simulink model "ovap_sim"  (R2025a)
settings: Solver=FixedStepAuto  StartTime=0.0  StopTime=100  FixedStep=0.002  RelTol=1e-3
undefined symbols (not defined in the file): X, Y, Z
libraries: sm_lib x88, nesl_utility x45, simulink_extras x31, slpidlib x8
(part 4 of 5)

== matlab function ovap_sim/3_Actuator_Dynamics/MATLAB Function ==
  settings: updateMethod=DISCRETE  sampleTime=0.002
  data: cmd_thrust input; phys_thrust output; cmd_alpha input; cmd_beta input; dt input; tau_motor input; tau_servo input; rate_lim input; lim_tilt input; phys_alpha output; phys_beta output
function [phys_thrust, phys_alpha, phys_beta] = Actuator_Dynamics(cmd_thrust, cmd_alpha, cmd_beta, ...
    dt, tau_motor, tau_servo, rate_lim, lim_tilt)
% =========================================================================
% Tên hàm: Actuator_Dynamics (Động lực học Cơ cấu chấp hành)
% Chức năng: Đóng vai trò làm "Bộ lọc Hiện thực". Biến các mệnh lệnh toán học
%            tức thời (cmd_) thành phản ứng vật lý thực tế có độ trễ (phys_).
% Nguyên lý: Mô phỏng Quán tính Rotor (First-Order Lag) và Giới hạn bánh răng
%            Servo (Rate Limit & Saturation).
% =========================================================================

    % ---------------------------------------------------------------------
    % 1. BỘ NHỚ VẬT LÝ (PERSISTENT STATE)
    % Ý nghĩa: Trong thế giới thực, một vật thể không thể dịch chuyển tức thời
    % từ trạng thái A sang B. Trạng thái tiếp theo luôn phụ thuộc vào trạng
    % thái hiện tại. Biến persistent đóng vai trò là "quán tính" của hệ thống.
    % ---------------------------------------------------------------------
    persistent prev_thrust prev_alpha prev_beta
    
    % Khởi tạo trạng thái đứng im khi bắt đầu bật điện (t = 0)
    if isempty(prev_thrust)
        prev_thrust = zeros(8,1); % Lực đẩy 8 motor = 0 N
        prev_alpha  = zeros(4,1); % Góc gật 4 ngàm = 0 rad
        prev_beta   = zeros(4,1); % Góc lật 4 ngàm = 0 rad
    end

    % ---------------------------------------------------------------------
    % 2. ĐỘNG LỰC HỌC ĐỘNG CƠ (MOTOR DYNAMICS - THUẬT TOÁN PT1)
    % Bản chất: Lõi chuông motor và cánh quạt 7-inch có khối lượng (Inertia).
    % Khi ESC bơm dòng điện, từ trường sinh ra momen xoắn để thắng sức ỳ này.
    % Thời gian để đạt được lực đẩy yêu cầu được đặc trưng bởi tau_motor (Ví dụ: 0.03s).
    % ---------------------------------------------------------------------
    % Tính hệ số lọc (Alpha) của bộ lọc thông thấp bậc 1 (First-Order Low-pass)
    % Hệ số này quyết định motor "bám theo" lệnh nhanh hay chậm dựa trên bước nhảy dt.
    alpha_m = dt / (tau_motor + dt);
    
    % Lực đẩy thực tế sẽ bám đuổi (chasing) lệnh yêu cầu.
    % Nếu lệch càng nhiều (cmd - prev lớn), motor tăng tốc càng mạnh.
    thrust_next = prev_thrust + alpha_m * (cmd_thrust - prev_thrust);
    
    % Giới hạn vật lý: Động cơ BLDC gắn cánh quạt tĩnh không thể tạo lực đẩy âm
    % (Trừ khi ESC dùng chế độ 3D đảo chiều quay, nhưng OVAP-X1 không dùng).
    phys_thrust = max(0, thrust_next); 

    % ---------------------------------------------------------------------
    % 3. ĐỘNG LỰC HỌC SERVO (SERVO DYNAMICS - LAG & RATE LIMIT)
    % Bản chất: Servo xịn như KST có mạch điều khiển bên trong (gây trễ tau_servo),
    % và hộp số bánh răng kim loại có tốc độ quay tối đa (rate_lim, ví dụ: 300 deg/s).
    % ---------------------------------------------------------------------
    % Hệ số độ trễ của mạch điện điều khiển Servo
    alpha_s = dt / (tau_servo + dt);
    
    % GIỚI HẠN TỐC ĐỘ (Rate Limit): Quãng đường góc lớn nhất (rad) mà bánh răng 
    % cơ khí có thể quét được trong khoảng thời gian siêu ngắn dt (0.002s).
    max_step = rate_lim * dt; 
    
    % ================= KÊNH ALPHA (NGÀM GẬP PITCH) =================
    % 3.1. Tính vị trí lý tưởng mà Servo "muốn" đạt tới (chỉ xét độ trễ mạch điện)
    ideal_alpha = prev_alpha + alpha_s * (cmd_alpha - prev_alpha); 
    
    % 3.2. Tính quãng đường góc cần di chuyển trong bước này
    delta_alpha = ideal_alpha - prev_alpha;
    
    % 3.3. ÁP DỤNG NÚT THẮT CỔ CHAI CƠ KHÍ (Rate Clamping)
    % Nếu lệnh bắt Servo quay nhanh hơn khả năng của motor bên trong, 
    % nó sẽ bị "nghẽn" lại và chỉ xoay được đúng bằng max_step.
    delta_alpha = max(min(delta_alpha, max_step), -max_step);      
    
    % 3.4. Vị trí thực tế Servo đạt được sau 1 bước dt
    phys_alpha = prev_alpha + delta_alpha;
    
    % 3.5. VA CHẠM CƠ KHÍ (Hard Stop / Saturation)
    phys_alpha = max(min(phys_alpha, lim_tilt), -lim_tilt);        
    
    % ================= KÊNH BETA (NGÀM LẬT ROLL) =================
    % (Áp dụng chính xác các quy luật vật lý tương tự như Kênh Alpha)
    ideal_beta = prev_beta + alpha_s * (cmd_beta - prev_beta);     
    delta_beta = ideal_beta - prev_beta;
    delta_beta = max(min(delta_beta, max_step), -max_step);        
    
    phys_beta = prev_beta + delta_beta;
    phys_beta = max(min(phys_beta, lim_tilt), -lim_tilt);          

    % ---------------------------------------------------------------------
    % 4. CẬP NHẬT TRẠNG THÁI (TIME MARCHING)
    % Ý nghĩa: Dòng thời gian trôi đi. Hiện tại của vòng lặp này sẽ trở thành 
    % quá khứ (prev_) cho vòng lặp tích phân tiếp theo.
    % ---------------------------------------------------------------------
    prev_thrust = phys_thrust;
    prev_alpha  = phys_alpha;
    prev_beta   = phys_beta;
end

== matlab function ovap_sim/2_Flight_Control_System/PID - 1/MATLAB Function1 ==
  data: ax_world input; cmd_hw_alpha output; ay_world input; cmd_thrust_z input; cmd_effort_roll input; cmd_effort_pitch input; cmd_effort_yaw input; yaw input; pitch input; roll input; phys_alpha_hw input; phys_beta_hw input; m input; g input; dir_alpha input; dir_beta input; lim_alpha input; lim_beta input; cmd_hw_beta output; cmd_thrust output; R_mat input; eta_c input; lam_c input; c_q input; dir_top input; max_thrust input
function [cmd_hw_alpha, cmd_hw_beta, cmd_thrust] = OVAP_Unified_Mixer(...
    ax_world, ay_world, ...                             
    cmd_thrust_z, cmd_effort_roll, cmd_effort_pitch, cmd_effort_yaw, ... 
    yaw, pitch, roll, ...                               
    phys_alpha_hw, phys_beta_hw, ...                    
    m, g, ...                                           
    dir_alpha, dir_beta, lim_alpha, lim_beta, ...
    R_mat, eta_c, lam_c, c_q, dir_top, max_thrust)            
% =========================================================================
% BỘ ĐIỀU KHIỂN CHẤP HÀNH TỔNG HỢP OVAP (UNIFIED ACTUATION MIXER) V7.5
% Kiến trúc: SYNCHRONOUS VECTORING + FEEDFORWARD ATTITUDE ASSIST
% [CẬP NHẬT MỚI]: Auto-Routing dựa trên Tọa độ Ma trận Hình học (R_mat).
% =========================================================================
    
    phys_alpha_hw = phys_alpha_hw(:); 
    phys_beta_hw  = phys_beta_hw(:);
    dir_alpha     = dir_alpha(:);
    dir_beta      = dir_beta(:);
    dir_top       = dir_top(:); 
    
    % =====================================================================
    % [HỆ SỐ HỖ TRỢ TƯ THẾ (FEEDFORWARD GAINS)]
    % =====================================================================
    K_assist_pitch = 0; 
    K_assist_roll  = 0; 
    lim_assist     = 0.17; 
    
    % =====================================================================
    % [TRIGGER BÁN CẦU] - NHẬN DIỆN MÁY BAY LẬT ÚP
    % =====================================================================
    inv_x = sign(cos(pitch) + eps);  
    inv_y = sign(cos(roll)  + eps);
    
    % =====================================================================
    % PHÂN VÙNG 1: ĐỒNG BỘ PHẢN HỒI (HARDWARE TO MATH)
    % =====================================================================
    math_alpha_fb = phys_alpha_hw ./ dir_alpha;  
    math_beta_fb  = phys_beta_hw  ./ dir_beta;  
    
    % =====================================================================
    % PHÂN VÙNG 2: BỘ TÍNH TOÁN VỊ TRÍ & TÍCH HỢP HỖ TRỢ TƯ THẾ
    % =====================================================================
    ax_heading = ax_world * cos(yaw) + ay_world * sin(yaw);   
    ay_heading = -ax_world * sin(yaw) + ay_world * cos(yaw); 
    
    ax_body_sync = ax_heading; 
    ay_body_sync = ay_heading; 
    
    ratio_x = max(min(ax_body_sync / g, 0.99), -0.99); 
    ratio_y = max(min(ay_body_sync / g, 0.99), -0.99); 
    
    alpha_base_array = zeros(4,1) + asin(ratio_x);
    beta_base_array  = zeros(4,1) + asin(ratio_y);  
    
    assist_pitch = max(min(cmd_effort_pitch * K_assist_pitch, lim_assist), -lim_assist);
    assist_roll  = max(min(cmd_effort_roll  * K_assist_roll,  lim_assist), -lim_assist);
    
    cmd_math_alpha = alpha_base_array + pitch + assist_pitch; 
    cmd_math_beta  = beta_base_array  - roll  + assist_roll;  
    
    cmd_math_alpha = atan2(sin(cmd_math_alpha), cos(cmd_math_alpha));
    cmd_math_beta  = atan2(sin(cmd_math_beta),  cos(cmd_math_beta));
    
    % =====================================================================
    % PHÂN VÙNG 3: BỘ PHÂN BỔ NGÀM VẬT LÝ (HARDWARE SERVO MAPPER)
    % =====================================================================
    cmd_hw_alpha = cmd_math_alpha .* dir_alpha; 
    cmd_hw_beta  = cmd_math_beta  .* dir_beta;  
    
    cmd_hw_alpha = max(min(cmd_hw_alpha, lim_alpha), -lim_alpha); 
    cmd_hw_beta  = max(min(cmd_hw_beta,  lim_beta),  -lim_beta);  
    
    % =====================================================================
    % PHÂN VÙNG 4: BỘ TRỘN ĐỘNG CƠ (R-CRM MOTOR MIXER TƯỜNG MINH)
    % =====================================================================
    global_alpha = math_alpha_fb - pitch;  
    global_beta  = math_beta_fb  + roll;
    
    mean_global_alpha = mean(abs(global_alpha)); 
    mean_global_beta  = mean(abs(global_beta));  
    
    total_z_req = cmd_thrust_z + m * g;
    T_base = (total_z_req / (cos(mean_global_alpha) * cos(mean_global_beta))) / 4;
    
    K_cross_pitch = 0.0; 
    K_cross_roll = 0.0; 
    pitch_parasitic = K_cross_pitch * sin(mean(math_alpha_fb)); 
    roll_parasitic  = K_cross_roll  * sin(mean(math_beta_fb));  
    
    real_cmd_pitch = (cmd_effort_pitch - pitch_parasitic) * inv_x;
    real_cmd_roll  = (cmd_effort_roll  - roll_parasitic)  * inv_y;
    
    % [CẬP NHẬT]: Trích xuất dist_x, dist_y (Vẫn lấy từ R_mat để dễ chỉnh kích thước)
    dist_x = abs(R_mat(1, 1));
    dist_y = abs(R_mat(1, 2));
    
    d_pitch = real_cmd_pitch / (4 * dist_x);
    d_roll  = real_cmd_roll  / (4 * dist_y);
    d_yaw   = cmd_effort_yaw / 4; 
    
    cmd_thrust = zeros(8,1); 
    limit_thrust = max_thrust(end);

    % -------------------------------------------------------------------------
    % ARM 1: FRONT-RIGHT (FR) 
    % Gốc: math_thrust(1) = base + pitch - roll + yaw (Top)
    %      math_thrust(6) = base + pitch - roll - yaw (Bot)
    % -------------------------------------------------------------------------
    T_arm1  = T_base + d_pitch - d_roll;
    dT_1    = d_yaw / c_q; % Dấu dương để T_top tăng (+yaw), T_bot giảm (-yaw)
    
    T_bot_6 = (T_arm1 - dT_1) / (eta_c + lam_c);
    T_top_1 = T_arm1 - eta_c * T_bot_6;
    
    if T_bot_6 < 0, T_bot_6 = 0; T_top_1 = T_arm1; end
    if T_top_1 < 0, T_top_1 = 0; T_bot_6 = T_arm1 / eta_c; end
    
    cmd_thrust(1) = min(max(T_top_1, 0), limit_thrust); % Top
    cmd_thrust(6) = min(max(T_bot_6, 0), limit_thrust); % Bot

    % -------------------------------------------------------------------------
    % ARM 2: FRONT-LEFT (FL) 
    % Gốc: math_thrust(2) = base + pitch + roll - yaw (Top)
    %      math_thrust(5) = base + pitch + roll + yaw (Bot)
    % -------------------------------------------------------------------------
    T_arm2  = T_base + d_pitch + d_roll;
    dT_2    = -d_yaw / c_q; % Dấu âm để T_top giảm (-yaw), T_bot tăng (+yaw)
    
    T_bot_5 = (T_arm2 - dT_2) / (eta_c + lam_c);
    T_top_2 = T_arm2 - eta_c * T_bot_5;
    
    if T_bot_5 < 0, T_bot_5 = 0; T_top_2 = T_arm2; end
    if T_top_2 < 0, T_top_2 = 0; T_bot_5 = T_arm2 / eta_c; end
    
    cmd_thrust(2) = min(max(T_top_2, 0), limit_thrust); % Top
    cmd_thrust(5) = min(max(T_bot_5, 0), limit_thrust); % Bot

    % -------------------------------------------------------------------------
    % ARM 3: REAR-LEFT (RL) 
    % Gốc: math_thrust(3) = base - pitch + roll + yaw (Top)
    %      math_thrust(8) = base - pitch + roll - yaw (Bot)
    % -------------------------------------------------------------------------
    T_arm3  = T_base - d_pitch + d_roll;
    dT_3    = d_yaw / c_q; % Dấu dương để T_top tăng (+yaw), T_bot giảm (-yaw)
    
    T_bot_8 = (T_arm3 - dT_3) / (eta_c + lam_c);
    T_top_3 = T_arm3 - eta_c * T_bot_8;
    
    if T_bot_8 < 0, T_bot_8 = 0; T_top_3 = T_arm3; end
    if T_top_3 < 0, T_top_3 = 0; T_bot_8 = T_arm3 / eta_c; end
    
    cmd_thrust(3) = min(max(T_top_3, 0), limit_thrust); % Top
    cmd_thrust(8) = min(max(T_bot_8, 0), limit_thrust); % Bot

    % -------------------------------------------------------------------------
    % ARM 4: REAR-RIGHT (RR) 
    % Gốc: math_thrust(4) = base - pitch - roll - yaw (Top)
    %      math_thrust(7) = base - pitch - roll + yaw (Bot)
    % -------------------------------------------------------------------------
    T_arm4  = T_base - d_pitch - d_roll;
    dT_4    = -d_yaw / c_q; % Dấu âm để T_top giảm (-yaw), T_bot tăng (+yaw)
    
    T_bot_7 = (T_arm4 - dT_4) / (eta_c + lam_c);
    T_top_4 = T_arm4 - eta_c * T_bot_7;
    
    if T_bot_7 < 0, T_bot_7 = 0; T_top_4 = T_arm4; end
    if T_top_4 < 0, T_top_4 = 0; T_bot_7 = T_arm4 / eta_c; end
    
    cmd_thrust(4) = min(max(T_top_4, 0), limit_thrust); % Top
    cmd_thrust(7) = min(max(T_bot_7, 0), limit_thrust); % Bot
end

== matlab function ovap_sim/2_Flight_Control_System/PID - 1/PID ==
  settings: updateMethod=DISCRETE
  data: sp_pos input; sp_vel input; cur_pos input; cur_vel input; kp_pos input; kp_vel input; ki_vel input; kd_vel input; sp_euler input; sp_rate input; cur_euler input; cur_rate input; kp_att input; kp_rate input; ki_rate input; kd_rate input; enable_pos input; enable_att input; cmd_pos output; dt input; cmd_att output
function [cmd_pos, cmd_att] = Main_PID_Controller(...
    sp_pos, sp_vel, cur_pos, cur_vel, kp_pos, kp_vel, ki_vel, kd_vel, ...
    sp_euler, sp_rate, cur_euler, cur_rate, kp_att, kp_rate, ki_rate, kd_rate, ...
    enable_pos, enable_att, dt)
% =========================================================================
% BỘ ĐIỀU KHIỂN TRUNG TÂM (CASCADED PID) - CÓ TÍCH HỢP CÔNG TẮC DEBUG
% =========================================================================

    % Khởi tạo bộ nhớ cho khâu I (Integral) và khâu D (Derivative)
    persistent int_vel prev_err_vel int_rate prev_err_rate
    if isempty(int_vel)
        int_vel = zeros(3,1);
        prev_err_vel = zeros(3,1);
        int_rate = zeros(3,1);
        prev_err_rate = zeros(3,1);
    end

    % Đảm bảo vector cột
    sp_pos = sp_pos(:); sp_vel = sp_vel(:); cur_pos = cur_pos(:); cur_vel = cur_vel(:);
    sp_euler = sp_euler(:); sp_rate = sp_rate(:); cur_euler = cur_euler(:); cur_rate = cur_rate(:);
    
    cmd_pos = zeros(3,1); % [cmd_x; cmd_y; cmd_z]
    cmd_att = zeros(3,1); % [cmd_roll; cmd_pitch; cmd_yaw]

    % =========================================================
    % 1. LUỒNG ĐIỀU KHIỂN VỊ TRÍ (POSITION -> VELOCITY)
    % =========================================================
    if enable_pos == 1
        % Vòng ngoài (P): Tính vận tốc mong muốn dựa trên sai số vị trí
        err_pos = sp_pos - cur_pos;
        target_vel = sp_vel + kp_pos(:) .* err_pos; % Có Feed-forward vận tốc
        
        % Vòng trong (PID): Tính lực/gia tốc mong muốn dựa trên sai số vận tốc
        err_vel = target_vel - cur_vel;
        
        int_vel = int_vel + err_vel * dt;
        % Chống bão hòa khâu I (Windup Limit cơ bản)
        int_vel = max(min(int_vel, 10), -10); 
        
        deriv_vel = (err_vel - prev_err_vel) / dt;
        prev_err_vel = err_vel;
        
        % Lệnh xuất ra: Lực ảo (cmd_x, cmd_y, cmd_z)
        cmd_pos = kp_vel(:) .* err_vel + ki_vel(:) .* int_vel + kd_vel(:) .* deriv_vel;
    else
        % NẾU TẮT VỊ TRÍ: Xóa sạch khâu I để không tích lũy rác, lệnh = 0
        int_vel = zeros(3,1);
        cmd_pos = zeros(3,1); 
        % Lưu ý: cmd_z = 0 ở đây không làm UAV rớt, vì lực Hover cơ bản 
        % sẽ được cộng vào ở khối Mixer phía sau.
    end

    % =========================================================
    % 2. LUỒNG ĐIỀU KHIỂN TƯ THẾ (ATTITUDE -> RATE)
    % =========================================================
    if enable_att == 1
        % Sai số góc Euler (Xử lý gói góc Yaw trong khoảng [-pi, pi])
        err_euler = sp_euler - cur_euler;
        err_euler(3) = atan2(sin(err_euler(3)), cos(err_euler(3)));
        
        % Vòng ngoài (P): Tính tốc độ xoay mong muốn
        target_rate = sp_rate + kp_att(:) .* err_euler; % Feed-forward rate
        
        % Vòng trong (PID): Tính momen mong muốn
        err_rate = target_rate - cur_rate;
        
        int_rate = int_rate + err_rate * dt;
        % Chống bão hòa khâu I
        int_rate = max(min(int_rate, 5), -5);
        
        deriv_rate = (err_rate - prev_err_rate) / dt;
        prev_err_rate = err_rate;
        
        % Lệnh xuất ra: Momen ảo (cmd_roll, cmd_pitch, cmd_yaw)
        cmd_att = kp_rate(:) .* err_rate + ki_rate(:) .* int_rate + kd_rate(:) .* deriv_rate;
    else
        % NẾU TẮT TƯ THẾ: Máy bay sẽ trôi lơ lửng, không cố gắng giữ thăng bằng
        int_rate = zeros(3,1);
        cmd_att = zeros(3,1);
    end
end

== matlab function ovap_sim/2_Flight_Control_System/WPIN - 2/MATLAB Function ==
  data: math_thrust input; cmd_thrust_px4 output; cmd_math_alpha input; cmd_math_beta input; phys_alpha_hw input; phys_beta_hw input; dir_alpha input; dir_beta input; lim_alpha input; lim_beta input; cmd_hw_alpha output; cmd_hw_beta output; math_alpha_fb output; math_beta_fb output
function [cmd_thrust_px4, cmd_hw_alpha, cmd_hw_beta, math_alpha_fb, math_beta_fb] = Hardware_Mapper(...
    math_thrust, cmd_math_alpha, cmd_math_beta, phys_alpha_hw, phys_beta_hw, ...
    dir_alpha, dir_beta, lim_alpha, lim_beta)
% KHỐI CHUYỂN HÓA 2 CHIỀU: MAP SENSOR VÀ MAP ACTUATOR

    % ---------------------------------------------------------
    % 1. ĐẦU VÀO: Đọc góc thật từ Actuator -> Chuyển thành góc Toán học
    % (Cấp math_alpha_fb, math_beta_fb ngược lại cho khối WPIN_Core)
    % ---------------------------------------------------------
    math_alpha_fb = phys_alpha_hw(:) .* dir_alpha(:);
    math_beta_fb  = phys_beta_hw(:)  .* dir_beta(:);
    
    % ---------------------------------------------------------
    % 2. ĐẦU RA ACTUATOR: Góc lý tưởng -> Góc Servo thật & Saturation
    % ---------------------------------------------------------
    cmd_hw_alpha = cmd_math_alpha(:) .* dir_alpha(:);
    cmd_hw_beta  = cmd_math_beta(:)  .* dir_beta(:);
    
    cmd_hw_alpha = max(min(cmd_hw_alpha, lim_alpha), -lim_alpha);
    cmd_hw_beta  = max(min(cmd_hw_beta,  lim_beta),  -lim_beta);
    
    % ---------------------------------------------------------
    % 3. ĐẦU RA ESC: Map Thrust M1->M8 theo đúng chuẩn PX4 Octorotor Coaxial
    % math_thrust(1:8) đang chứa: [Top1, Bot1, Top2, Bot2, Top3, Bot3, Top4, Bot4]
    % ---------------------------------------------------------
    cmd_thrust_px4 = zeros(8,1);
    
    % Arm 1 (FR)
    cmd_thrust_px4(1) = math_thrust(1); % M1: Top FR (CCW)
    cmd_thrust_px4(6) = math_thrust(2); % M6: Bot FR (CW)
    
    % Arm 2 (RL)
    cmd_thrust_px4(3) = math_thrust(3); % M3: Top RL (CCW)
    cmd_thrust_px4(8) = math_thrust(4); % M8: Bot RL (CW)
    
    % Arm 3 (FL)
    cmd_thrust_px4(2) = math_thrust(5); % M2: Top FL (CW)
    cmd_thrust_px4(5) = math_thrust(6); % M5: Bot FL (CCW)
    
    % Arm 4 (RR)
    cmd_thrust_px4(4) = math_thrust(7); % M4: Top RR (CW)
    cmd_thrust_px4(7) = math_thrust(8); % M7: Bot RR (CCW)
end

== matlab function ovap_sim/2_Flight_Control_System/PID - 1/Servo Controll ==
  data: cmd_x input; cmd_y input; cmd_pitch input; cmd_roll input; cmd_math_alpha output; cmd_math_beta output; dt input; max_tilt input; speed_gain_pos input; speed_gain_att input
function [cmd_math_alpha, cmd_math_beta] = Servo_Sub_Controller(cmd_x, cmd_y, cmd_pitch, cmd_roll, dt, max_tilt, speed_gain_pos, speed_gain_att)
% =========================================================================
% BỘ ĐIỀU KHIỂN PHỤ SERVO (VELOCITY-BASED INTEGRATION)
% Chức năng: Nhận lệnh từ PID chính -> Quy đổi thành Tốc độ xoay -> Tích 
% phân ra góc lý tưởng. Đảm bảo xoay mượt mà, không giật cục.
% =========================================================================

    % Khởi tạo bộ nhớ lưu góc hiện tại của Servo (đóng vai trò Khâu Tích phân)
    persistent alpha_state beta_state
    if isempty(alpha_state)
        alpha_state = zeros(4,1);
        beta_state  = zeros(4,1);
    end

    % Đảm bảo an toàn dữ liệu
    cmd_x = cmd_x(1); cmd_y = cmd_y(1); 
    cmd_pitch = cmd_pitch(1); cmd_roll = cmd_roll(1);

    % =========================================================
    % 1. TÍNH TỐC ĐỘ XOAY SERVO (RATE)
    % Lệnh lớn -> Tốc độ băm nhanh. Lệnh nhỏ -> Tốc độ rà chậm.
    % =========================================================
    % Trục X (tiến/lùi) và Pitch tác động lên ngàm Alpha
    % (Dấu +/- ở đây tùy thuộc vào quy ước hệ trục toán học của bạn, có thể đổi lại khi test)
    rate_alpha = (speed_gain_pos * cmd_x) + (speed_gain_att * cmd_pitch); 
    
    % Trục Y (trái/phải) và Roll tác động lên ngàm Beta
    rate_beta  = (speed_gain_pos * cmd_y) + (speed_gain_att * cmd_roll);

    % =========================================================
    % 2. TÍCH PHÂN VẬN TỐC THÀNH GÓC (XOAY DẦN ĐỀU)
    % Vị trí góc mới = Vị trí góc cũ + (Vận tốc xoay * dt)
    % Cả 4 ngàm nhận chung 1 lệnh toán học đồng nhất.
    % =========================================================
    alpha_state = alpha_state + rate_alpha * dt * ones(4,1);
    beta_state  = beta_state  + rate_beta  * dt * ones(4,1);

    % =========================================================
    % 3. GIỚI HẠN GÓC GẬP (SATURATION)
    % Khóa trần góc xoay để Servo không bẻ gãy khung carbon.
    % Ví dụ: max_tilt = 30 độ (0.52 rad)
    % =========================================================
    alpha_state = max(min(alpha_state, max_tilt), -max_tilt);
    beta_state  = max(min(beta_state, max_tilt), -max_tilt);

    % Xuất góc toán học thuần túy (Truyền đi cho Hardware Mapper)
    cmd_math_alpha = alpha_state;
    cmd_math_beta  = beta_state;
end

== matlab function ovap_sim/1_Mission_Planner/MATLAB Function1 ==
  settings: updateMethod=DISCRETE
  data: t input; v_max input; a_max input; w_max input; alpha_max input; dt input; sp_pos output; sp_vel output; sp_acc output; sp_euler output; sp_rate output; g input; lim_tilt input; rate_lim_tilt input
function [sp_pos, sp_vel, sp_acc, sp_euler, sp_rate] = Mission_Planner(...
    t, v_max, a_max, w_max, alpha_max, dt, ...
    g, lim_tilt, rate_lim_tilt) % [MỚI] Các đầu vào ràng buộc phần cứng
% =========================================================================
% KINEMATIC TRAJECTORY PLANNER (Bộ tạo quỹ đạo động học nhận biết Actuator)
% Cập nhật: Chuyển các giới hạn phần cứng thành Cổng đầu vào (Input Ports)
% =========================================================================

    % Khởi tạo bộ nhớ cho các khâu Tích phân
    persistent traj_pos traj_vel traj_acc traj_euler traj_rate traj_rate_dot
    if isempty(traj_pos)
        traj_pos = zeros(3,1); traj_vel = zeros(3,1); traj_acc = zeros(3,1);
        traj_euler = zeros(3,1); traj_rate = zeros(3,1); traj_rate_dot = zeros(3,1);
    end
    planner_mode = 1;
    % =====================================================================
    % 1. MISSION MANAGER (Tạo tọa độ mục tiêu thô)
    % =====================================================================
    target_pos   = [0; 0; 0];
    target_euler = [0; 0; 0];
    
    if t < 5.0
        target_pos = [0; 0; 5.0]; 
    elseif t < 10.0
        target_pos = [0; 0; 5.0]; 
    elseif t < 20.0
        target_pos = [5; 0; 10.0]; 
    elseif t < 30.0
        target_pos = [-10; 0; 10.0]; 
    else
        target_pos = [20; 0; 25.0]; 
    end
    
    % Chuyển đổi sang Radian và Cuộn Yaw về chuẩn [-pi, pi]
    target_euler = target_euler * (pi / 180);
    target_euler(3) = mod(target_euler(3) + pi, 2*pi) - pi;

    % =====================================================================
    % 2. TRAJECTORY PLANNER (Bộ tạo quỹ đạo 2 Chế độ)
    % =====================================================================
    if planner_mode == 0
        % -----------------------------------------------------------------
        % [MODE 0]: HÀM NẤC (TUNE PID)
        % -----------------------------------------------------------------
        traj_pos   = target_pos;
        traj_vel   = zeros(3,1);
        traj_acc   = zeros(3,1);
        traj_euler = target_euler;
        traj_rate  = zeros(3,1);
        traj_rate_dot = zeros(3,1);
        
    else
        % -----------------------------------------------------------------
        % [MODE 1]: LÀM MƯỢT ĐỘNG HỌC CÓ RÀNG BUỘC PHẦN CỨNG (S-CURVE)
        % -----------------------------------------------------------------
        k_pos_smooth = 1.0; 
        k_att_smooth = 1.0; 
        
        % --- ĐỒNG BỘ GIỚI HẠN VẬT LÝ ---
        % 1. Gia tốc ngang tối đa (Phụ thuộc vào góc nghiêng ngàm Servo lớn nhất)
        a_max_hw = [g * sin(lim_tilt); 
                    g * sin(lim_tilt); 
                    a_max(3)]; % Trục Z tạm dùng giới hạn mềm
                    
        % 2. Độ giật tối đa - Max Jerk (Phụ thuộc vào Tốc độ xoay Servo)
        jerk_max_hw = [g * rate_lim_tilt; 
                       g * rate_lim_tilt; 
                       50.0]; % Trục Z motor đáp ứng rất nhanh
                       
        % 3. Gia tốc góc lật tối đa (Phụ thuộc vào Tốc độ bẻ Servo)
        alpha_max_hw = [rate_lim_tilt; 
                        rate_lim_tilt; 
                        alpha_max(3)];

        % --- XỬ LÝ QUỸ ĐẠO TỊNH TIẾN (POSITION) ---
        for i = 1:3
            % Tính Vận tốc mong muốn (S-Curve thô)
            pos_err = target_pos(i) - traj_pos(i);
            v_target = v_max(i) * tanh((k_pos_smooth * pos_err) / v_max(i));
            
            % Tính Gia tốc lý thuyết cần thiết
            a_req_raw = (v_target - traj_vel(i)) / dt;
            
            % BƯỚC 1: Ràng buộc Tốc độ bẻ ngàm (Chặn Jerk)
            jerk_req = (a_req_raw - traj_acc(i)) / dt;
            jerk_req = max(min(jerk_req, jerk_max_hw(i)), -jerk_max_hw(i));
            
            % Tính ra Gia tốc khả thi (Sau khi đã chặn Jerk)
            a_req = traj_acc(i) + jerk_req * dt;
            
            % BƯỚC 2: Ràng buộc Biên độ bẻ ngàm (Chặn Accel)
            safe_a_max = min(a_max(i), a_max_hw(i));
            a_req = max(min(a_req, safe_a_max), -safe_a_max);
            
            % Tích phân Euler
            traj_acc(i) = a_req;
            traj_vel(i) = traj_vel(i) + traj_acc(i) * dt;
            traj_pos(i) = traj_pos(i) + traj_vel(i) * dt;
        end
        
        % --- XỬ LÝ QUỸ ĐẠO TƯ THẾ (ATTITUDE) ---
        for k = 1:3
            % Đi đường ngắn nhất cho Yaw
            if k == 3
                ang_err = target_euler(3) - traj_euler(3);
                ang_err = mod(ang_err + pi, 2*pi) - pi;
            else
                ang_err = target_euler(k) - traj_euler(k);
            end
            
            % Tốc độ góc mong muốn
            rate_target = w_max(k) * tanh((k_att_smooth * ang_err) / w_max(k));
            
            % Gia tốc góc lý thuyết
            alpha_req_raw = (rate_target - traj_rate(k)) / dt;
            
            % BƯỚC 3: Ràng buộc Gia tốc lật góc 
            safe_alpha_max = min(alpha_max(k), alpha_max_hw(k));
            alpha_req = max(min(alpha_req_raw, safe_alpha_max), -safe_alpha_max);
            
            % Tích phân
            traj_rate_dot(k) = alpha_req;
            traj_rate(k)     = traj_rate(k) + traj_rate_dot(k) * dt;
            traj_euler(k)    = traj_euler(k) + traj_rate(k) * dt;
            
            % Bọc góc Yaw sau khi tích phân
            if k == 3
                traj_euler(3) = mod(traj_euler(3) + pi, 2*pi) - pi;
            end
        end
    end
    
    % =====================================================================
    % 3. XUẤT TÍN HIỆU RA NGOÀI (Cho Bộ điều khiển vòng trong)
    % =====================================================================
    sp_pos   = traj_pos; 
    sp_vel   = traj_vel;
    sp_acc   = traj_acc;    % [ĐẦU RA MỚI] Dùng làm Feedforward Gia Tốc (Nếu cần)
    sp_euler = traj_euler; 
    sp_rate  = traj_rate;
end

== matlab function ovap_sim/2_Flight_Control_System/PID - 1/MATLAB Function2 ==
  data: out_x input; roll_sp output; out_y input; yaw_curr input; pitch_sp output
% function [roll_sp, pitch_sp] = Coordinate_Transform(out_x, out_y, yaw_curr)
%     % out_x, out_y: Lực đẩy mong muốn theo hệ World (NED)
%     % yaw_curr: Góc Yaw hiện tại (Radian)
% 
%     % 1. Xoay vector lệnh từ World sang Body
%     % Công thức ma trận xoay 2D
%     pitch_cmd_body = out_x * cos(yaw_curr) + out_y * sin(yaw_curr);
%     roll_cmd_body  = out_x * sin(yaw_curr) - out_y * cos(yaw_curr);
% 
%     % 2. Chuyển đổi sang Setpoint góc (Radian hoặc Độ)
%     % Lưu ý: +X world cần -Pitch body, +Y world cần +Roll body
%     pitch_sp = -pitch_cmd_body; 
%     roll_sp  =  roll_cmd_body;
% 
%     % 3. Giới hạn (Saturation) để đảm bảo an toàn
%     max_tilt = 0.17; % ~10 độ
%     pitch_sp = max(min(pitch_sp, max_tilt), -max_tilt);
%     roll_sp  = max(min(roll_sp,  max_tilt), -max_tilt);
% end
function [roll_sp, pitch_sp] = Coordinate_Transform(out_x, out_y, yaw_curr)
    % 1. Xoay vector từ World (NED) sang Body (Forward-Right)
    % Sử dụng ma trận xoay Rz(yaw) chuyển từ World sang Body:
    % [x_body]   [ cos(yaw)  sin(yaw)] [x_world]
    % [y_body] = [-sin(yaw)  cos(yaw)] [y_world]
    
    x_body_cmd =  out_x * cos(yaw_curr) + out_y * sin(yaw_curr);
    y_body_cmd = -out_x * sin(yaw_curr) + out_y * cos(yaw_curr);

    % 2. MAPPING SANG GÓC NGHIÊNG (Attitude Mapping)
    % Quy ước: 
    % - Để tiến tới (+x_body), cần chúi mũi (-Pitch)
    % - Để sang phải (+y_body), cần nghiêng phải (+Roll)
    
    pitch_sp = -x_body_cmd; 
    roll_sp  =  y_body_cmd; 
    
    % 3. Giới hạn (Saturation) 10 độ
    max_tilt = 0.17; 
    pitch_sp = max(min(pitch_sp, max_tilt), -max_tilt);
    roll_sp  = max(min(roll_sp,  max_tilt), -max_tilt);
end

== matlab function ovap_sim/2_Flight_Control_System/PID - 1/MATLAB Function3 ==
  data: ax_world input; cmd_hw_alpha output; ay_world input; cmd_thrust_z input; cmd_effort_roll input; cmd_effort_pitch input; cmd_effort_yaw input; yaw input; pitch input; roll input; phys_alpha_hw input; phys_beta_hw input; m input; g input; dir_alpha input; dir_beta input; lim_alpha input; lim_beta input; cmd_hw_beta output; cmd_thrust_px4 output
function [cmd_hw_alpha, cmd_hw_beta, cmd_thrust_px4] = OVAP_Unified_Mixer(...
    ax_world, ay_world, ...                             
    cmd_thrust_z, cmd_effort_roll, cmd_effort_pitch, cmd_effort_yaw, ... 
    yaw, pitch, roll, ...                               
    phys_alpha_hw, phys_beta_hw, ...                    
    m, g, ...                                           
    dir_alpha, dir_beta, lim_alpha, lim_beta)           
% =========================================================================
% BỘ ĐIỀU KHIỂN CHẤP HÀNH TỔNG HỢP OVAP (UNIFIED ACTUATION MIXER) V6.0
% Kiến trúc: SYNCHRONOUS VECTORING + FEEDFORWARD ATTITUDE ASSIST
% Điểm mới: Servo chủ động tham gia lật máy bay để triệt tiêu vọt lố Vị trí.
% =========================================================================
    
    phys_alpha_hw = phys_alpha_hw(:); 
    phys_beta_hw  = phys_beta_hw(:);
    dir_alpha     = dir_alpha(:);
    dir_beta      = dir_beta(:);

    % =====================================================================
    % [HỆ SỐ HỖ TRỢ TƯ THẾ (FEEDFORWARD GAINS)]
    % Quyết định mức độ Servo "phụ giúp" Motor lật máy bay.
    % Bắt đầu tune từ số nhỏ (0.1 - 0.3) để xem chiều tác động.
    % Nếu Servo bẻ ngược hướng lật mong muốn, hãy đổi dấu thành số âm.
    % =====================================================================
    K_assist_pitch = 0; % Bù chéo từ lệnh Pitch sang Servo Alpha
    K_assist_roll  = 0; % Bù chéo từ lệnh Roll sang Servo Beta

    % =====================================================================
    % [TRIGGER BÁN CẦU] - NHẬN DIỆN MÁY BAY LẬT ÚP
    % Chỉ dùng cho Motor Mixer (Thái độ).
    % =====================================================================
    inv_x = sign(cos(pitch) + eps);  
    inv_y = sign(cos(roll)  + eps);

    % =====================================================================
    % PHÂN VÙNG 1: ĐỒNG BỘ PHẢN HỒI (HARDWARE TO MATH)
    % =====================================================================
    math_alpha_fb = phys_alpha_hw ./ dir_alpha;  
    math_beta_fb  = phys_beta_hw  ./ dir_beta;  

    % =====================================================================
    % PHÂN VÙNG 2: BỘ TÍNH TOÁN VỊ TRÍ & TÍCH HỢP HỖ TRỢ TƯ THẾ
    % =====================================================================
    % 1. Xoay vector gia tốc PD từ hệ Earth sang hệ Heading
    ax_heading = ax_world * cos(yaw) + ay_world * sin(yaw);   
    ay_heading = -ax_world * sin(yaw) + ay_world * cos(yaw); 
    
    ax_body_sync = ax_heading; 
    ay_body_sync = ay_heading; 
    
    % Khóa gia tốc ngang không vượt quá trọng lực
    ratio_x = max(min(ax_body_sync / g, 0.99), -0.99); 
    ratio_y = max(min(ay_body_sync / g, 0.99), -0.99); 
    
    % 2. Tính toán góc Base đồng bộ
    alpha_base_sync = asin(ratio_x); 
    beta_base_sync  = asin(ratio_y); 
    
    alpha_base_array = zeros(4,1) + alpha_base_sync;
    beta_base_array  = zeros(4,1) + beta_base_sync;  
    
    % 3. [TÍCH HỢP FEEDFORWARD ASSIST & DECOUPLING]
    % Lệnh Servo = Bù Vị trí + Bù Tư Thế (Decouple) + Hỗ trợ lật (Assist)
    % cmd_effort_pitch/roll được trích xuất trực tiếp từ PID Thái độ để ép Servo bẻ sớm.
    cmd_math_alpha = alpha_base_array + pitch + (cmd_effort_pitch * K_assist_pitch); 
    cmd_math_beta  = beta_base_array  - roll  + (cmd_effort_roll  * K_assist_roll);  

    % cmd_math_alpha = alpha_base_array + (pitch * K_assist_pitch); 
    % cmd_math_beta  = beta_base_array  - (roll  * K_assist_roll);  
    
    % Wrap góc lượng giác đi đường ngắn nhất qua biên 360 độ
    cmd_math_alpha = atan2(sin(cmd_math_alpha), cos(cmd_math_alpha));
    cmd_math_beta  = atan2(sin(cmd_math_beta),  cos(cmd_math_beta));

    % =====================================================================
    % PHÂN VÙNG 3: BỘ PHÂN BỔ NGÀM VẬT LÝ (HARDWARE SERVO MAPPER)
    % =====================================================================
    cmd_hw_alpha = cmd_math_alpha .* dir_alpha; 
    cmd_hw_beta  = cmd_math_beta  .* dir_beta;  
    
    cmd_hw_alpha = max(min(cmd_hw_alpha, lim_alpha), -lim_alpha); 
    cmd_hw_beta  = max(min(cmd_hw_beta,  lim_beta),  -lim_beta);  

    % =====================================================================
    % PHÂN VÙNG 4: BỘ TRỘN ĐỘNG CƠ (MOTOR MIXER & Z-COMPENSATION)
    % =====================================================================
    % 1. GIẢI MÃ PHẢN HỒI GÓC GLOBAL
    % Lưu ý quan trọng: Dù Phân vùng 2 có chèn thêm Assist, ta KHÔNG CẦN trừ Assist ra ở đây.
    % Vì phản hồi thực tế (math_fb) đã bao gồm Assist rồi, ta chỉ việc giải mã góc thân (pitch/roll).
    global_alpha = math_alpha_fb - pitch;  
    global_beta  = math_beta_fb  + roll;
    
    mean_global_alpha = mean(abs(global_alpha)); 
    mean_global_beta  = mean(abs(global_beta));  
    
    total_z_req = cmd_thrust_z + m * g;
    base_thrust = (total_z_req / (cos(mean_global_alpha) * cos(mean_global_beta))) / 8;
    
    % 2. Xử lý Mô-men ký sinh do lệch tâm ngàm (Parasitic Torque)
    K_cross_pitch = 0; 
    K_cross_roll  = 0; 
    net_alpha = mean(math_alpha_fb);  
    net_beta  = mean(math_beta_fb);  
    pitch_parasitic = K_cross_pitch * sin(net_alpha); 
    roll_parasitic  = K_cross_roll  * sin(net_beta);  
    
    % 3. ÁP DỤNG LOGIC ĐẢO NHÁNH ĐỘNG CƠ
    real_cmd_pitch = (cmd_effort_pitch - pitch_parasitic) * inv_x;
    real_cmd_roll  = (cmd_effort_roll  - roll_parasitic)  * inv_y;
    real_cmd_yaw   = cmd_effort_yaw;
    
    math_thrust = zeros(8,1); 
    
    math_thrust(1) = base_thrust + real_cmd_pitch - real_cmd_roll + real_cmd_yaw; 
    math_thrust(6) = base_thrust + real_cmd_pitch - real_cmd_roll - real_cmd_yaw; 
    math_thrust(2) = base_thrust + real_cmd_pitch + real_cmd_roll - real_cmd_yaw; 
    math_thrust(5) = base_thrust + real_cmd_pitch + real_cmd_roll + real_cmd_yaw; 
    math_thrust(3) = base_thrust - real_cmd_pitch + real_cmd_roll + real_cmd_yaw; 
    math_thrust(8) = base_thrust - real_cmd_pitch + real_cmd_roll - real_cmd_yaw; 
    math_thrust(4) = base_thrust - real_cmd_pitch - real_cmd_roll - real_cmd_yaw; 
    math_thrust(7) = base_thrust - real_cmd_pitch - real_cmd_roll + real_cmd_yaw; 
    
    cmd_thrust_px4 = max(math_thrust, 0); 
end

== matlab function ovap_sim/2_Flight_Control_System/WPIN - 2/PID ==
  settings: updateMethod=DISCRETE
  data: sp_pos input; sp_vel input; sp_euler input; sp_rate input; tau_des output; State_X input; dt input; mass input; g input; pos_P input; vel_Kp input; vel_Ki input; vel_Kd input; max_vel input; max_acc input; att_P input; rate_Kp input; rate_Ki input; rate_Kd input; max_torque input
function tau_des = Flight_Controller(sp_pos, sp_vel, sp_euler, sp_rate, State_X, dt, mass, g, ...
                                     pos_P, vel_Kp, vel_Ki, vel_Kd, max_vel, max_acc, ...
                                     att_P, rate_Kp, rate_Ki, rate_Kd, max_torque)
% =========================================================================
% TÊN HÀM: Flight_Controller (Tương đương flight_main.m + position_ctrl + attitude_ctrl)
% CHỨC NĂNG: Điều khiển Vị trí và Tư thế TÁCH RỜI (Decoupled) cho Tilt-rotor.
% BẢN VÁ: Làm phẳng biến Persistent để tương thích 100% với Simulink Coder C/C++
% =========================================================================

    % ---------------------------------------------------------------------
    % 1. BỘ NHỚ VẬT LÝ TĨNH (THAY THẾ CHO STRUCT CELL ARRAY)
    % Khai báo dưới dạng Vector 3x1 để Simulink Coder hiểu được ngay lập tức
    % ---------------------------------------------------------------------
    persistent int_vel d_filt_vel prev_err_vel
    persistent int_rate d_filt_rate prev_err_rate
    
    if isempty(int_vel)
        int_vel       = zeros(3,1); 
        d_filt_vel    = zeros(3,1); 
        prev_err_vel  = zeros(3,1);
        int_rate      = zeros(3,1); 
        d_filt_rate   = zeros(3,1); 
        prev_err_rate = zeros(3,1);
    end

    % ---------------------------------------------------------------------
    % 2. ÉP KIỂU ĐẦU VÀO VÀ GIẢI MÃ TRẠNG THÁI
    % Ép toàn bộ thành Vector Cột (:), khắc phục triệt để lỗi Port Widths
    % ---------------------------------------------------------------------
    State_X = State_X(:);
    pos_earth = State_X(1:3);
    vel_body  = State_X(4:6); 
    euler     = State_X(7:9);
    rate_body = State_X(10:12);
    
    sp_pos   = sp_pos(:);   
    sp_euler = sp_euler(:); 
    
    % Ép các tham số giới hạn và Kp, Ki, Kd thành vector cột để tính toán Array-wise
    pos_P = pos_P(:); vel_Kp = vel_Kp(:); vel_Ki = vel_Ki(:); vel_Kd = vel_Kd(:);
    max_vel = max_vel(:); max_acc = max_acc(:);
    att_P = att_P(:); rate_Kp = rate_Kp(:); rate_Ki = rate_Ki(:); rate_Kd = rate_Kd(:);
    max_torque = max_torque(:);

    % --- Ma trận xoay (Body -> Earth) ---
    ph = euler(1); th = euler(2); ps = euler(3);
    R_b2e = [cos(th)*cos(ps), sin(ph)*sin(th)*cos(ps)-cos(ph)*sin(ps), cos(ph)*sin(th)*cos(ps)+sin(ph)*sin(ps);
             cos(th)*sin(ps), sin(ph)*sin(th)*sin(ps)+cos(ph)*cos(ps), cos(ph)*sin(th)*sin(ps)-sin(ph)*cos(ps);
            -sin(th),         sin(ph)*cos(th),                         cos(ph)*cos(th)];
            
    % Chuyển vận tốc đo được từ hệ Body sang Earth
    vel_earth = R_b2e * vel_body; 

    % =====================================================================
    % 3. VÒNG LẶP VỊ TRÍ (POSITION -> VELOCITY -> FORCE)
    % Sinh ra lực F_earth, sau đó chiếu về hệ Body (F_body_des)
    % =====================================================================
    pos_error = sp_pos - pos_earth;
    vel_sp_raw = pos_P .* pos_error; % KHÔNG cộng Feedforward để khớp 100% script gốc
    
    % Component-wise Velocity Saturation
    vel_sp = max(min(vel_sp_raw, max_vel), -max_vel);
    
    vel_error = vel_sp - vel_earth;
    acc_cmd_earth = zeros(3,1);
    
    for i = 1:3
        P = vel_Kp(i) * vel_error(i);
        
        % Khâu I với Dynamic Anti-windup
        int_vel(i) = int_vel(i) + vel_error(i) * dt;
        I_max = max_acc(i) * 0.5;
        int_vel(i) = max(min(int_vel(i), I_max/vel_Ki(i)), -I_max/vel_Ki(i));
        I = vel_Ki(i) * int_vel(i);
        
        % Khâu D với Low-pass filter 20Hz
        deriv_raw = (vel_error(i) - prev_err_vel(i)) / dt;
        alpha_f = dt / ((1.0 / (2*pi*20.0)) + dt);
        d_filt_vel(i) = alpha_f * deriv_raw + (1 - alpha_f) * d_filt_vel(i);
        D = vel_Kd(i) * d_filt_vel(i);
        
        acc_cmd_earth(i) = max(min(P + I + D, max_acc(i)), -max_acc(i));
        prev_err_vel(i) = vel_error(i);
    end
    
    % Bù trọng lực (hệ NED) và xoay vector lực về hệ Body
    F_earth_total = mass * (acc_cmd_earth - [0; 0; g]); 
    F_body_des = R_b2e' * F_earth_total;

    % =====================================================================
    % 4. VÒNG LẶP TƯ THẾ (ATTITUDE -> RATE -> MOMENT)
    % Hoàn toàn độc lập, chỉ quan tâm đến sp_euler từ Mission Planner
    % =====================================================================
    att_error = sp_euler - euler;
    att_error(3) = atan2(sin(att_error(3)), cos(att_error(3))); % Yaw wrapping
    
    rate_sp_raw = att_P .* att_error; % KHÔNG cộng Feedforward
    rate_error = rate_sp_raw - rate_body;
    
    M_body_des = zeros(3,1);
    
    for i = 1:3
        P = rate_Kp(i) * rate_error(i);
        
        % Khâu I với Dynamic Anti-windup
        int_rate(i) = int_rate(i) + rate_error(i) * dt;
        I_max = max_torque(i) * 0.5;
        int_rate(i) = max(min(int_rate(i), I_max/rate_Ki(i)), -I_max/rate_Ki(i));
        I = rate_Ki(i) * int_rate(i);
        
        % Khâu D với Low-pass filter 20Hz
        deriv_raw = (rate_error(i) - prev_err_rate(i)) / dt;
        alpha_f = dt / ((1.0 / (2*pi*20.0)) + dt);
        d_filt_rate(i) = alpha_f * deriv_raw + (1 - alpha_f) * d_filt_rate(i);
        D = rate_Kd(i) * d_filt_rate(i);
        
        M_body_des(i) = max(min(P + I + D, max_torque(i)), -max_torque(i));
        prev_err_rate(i) = rate_error(i);
    end

    % ---------------------------------------------------------------------
    % 5. ĐÓNG GÓI OUTPUT ĐỂ GỬI TỚI WPIN
    % Toàn bộ vector tau_des đã được chiếu chuẩn xác về hệ BODY
    % ---------------------------------------------------------------------
    tau_des = [F_body_des; M_body_des];
end

== matlab function ovap_sim/4_Vehicle_Dynamics_6DOF/MATLAB Function ==
  data: State_X input; dx output; phys_thrust input; phys_alpha input; phys_beta input; mass input; J input; invJ input; g input; r_mat input; h_eff input; kq input; coax_eff input; coax_tq_eff input; dir_top input; dir_alpha input; dir_beta input
function dx = Dynamics_6DOF(State_X, phys_thrust, phys_alpha, phys_beta, ...
    mass, J, invJ, g, r_mat, h_eff, kq, coax_eff, coax_tq_eff, dir_top, dir_alpha, dir_beta)
% PHƯƠNG TRÌNH ĐỘNG LỰC HỌC 6-DOF (Bản vá chống lỗi Dimension Mismatch)

    % 0. ÉP CỨNG KÍCH THƯỚC: Chặn đứng mọi rủi ro phình ma trận
    dx = zeros(12, 1);
    
    State_X = State_X(:);
    phys_thrust = phys_thrust(:); phys_alpha = phys_alpha(:); phys_beta = phys_beta(:);
    dir_top = dir_top(:); dir_alpha = dir_alpha(:); dir_beta = dir_beta(:);

    % 1. Giải mã Trạng thái
    vel_b = State_X(4:6);
    euler = State_X(7:9);
    rates = State_X(10:12);
    
    phi = euler(1); theta = euler(2); psi = euler(3);
    
    % 2. Lực & Momen Actuators
    F_act_b = zeros(3,1);
    M_act_b = zeros(3,1);
    
    for i = 1:4
        alpha = phys_alpha(i) * dir_alpha(i);
        beta  = phys_beta(i)  * dir_beta(i);
        sa = sin(alpha); ca = cos(alpha);
        sb = sin(beta);  cb = cos(beta);
        
        T_top = phys_thrust(i);
        T_bot = phys_thrust(i+4);
        T_i = T_top + T_bot * coax_eff;
        
        M_delta_i = dir_top(i) * kq * (T_top - coax_tq_eff * T_bot);
        
        vec_F_unit = [-sa * cb; sb; -ca * cb];
        F_i_local = T_i * vec_F_unit;
        
        R_s = [ ca,  sa*sb,  sa*cb;
                 0,     cb,    -sb;
               -sa,  ca*sb,  ca*cb];
        r_offset = R_s * [0; 0; -h_eff];
        r_total = r_mat(i,:)' + r_offset;
        
        M_force = [ r_total(2)*F_i_local(3) - r_total(3)*F_i_local(2);
                    r_total(3)*F_i_local(1) - r_total(1)*F_i_local(3);
                    r_total(1)*F_i_local(2) - r_total(2)*F_i_local(1) ];
        
        M_coax = M_delta_i * (-vec_F_unit);
        
        F_act_b = F_act_b + F_i_local;
        M_act_b = M_act_b + M_force + M_coax;
    end
    
    % 3. Môi trường
    g_b = g * [ -sin(theta); cos(theta)*sin(phi); cos(theta)*cos(phi) ];
    F_gravity_b = mass * g_b;
    
    Cd = [0.15; 0.15; 0.30]; 
    F_drag_b = -Cd .* vel_b;
    F_env_b = F_gravity_b + F_drag_b;
    
    % 4. Newton-Euler
    F_sum_b = F_act_b + F_env_b;
    M_sum_b = M_act_b; 
    
    cross_w_v = [ rates(2)*vel_b(3) - rates(3)*vel_b(2);
                  rates(3)*vel_b(1) - rates(1)*vel_b(3);
                  rates(1)*vel_b(2) - rates(2)*vel_b(1) ];
    acc_b = (F_sum_b / mass) - cross_w_v;
    
    Jw = J * rates;
    cross_w_Jw = [ rates(2)*Jw(3) - rates(3)*Jw(2);
                   rates(3)*Jw(1) - rates(1)*Jw(3);
                   rates(1)*Jw(2) - rates(2)*Jw(1) ];
    rate_dot = invJ * (M_sum_b - cross_w_Jw);
    
    % 5. Động học
    R_b2e = [ cos(theta)*cos(psi), sin(phi)*sin(theta)*cos(psi)-cos(phi)*sin(psi), cos(phi)*sin(theta)*cos(psi)+sin(phi)*sin(psi);
              cos(theta)*sin(psi), sin(phi)*sin(theta)*sin(psi)+cos(phi)*cos(psi), cos(phi)*sin(theta)*sin(psi)-sin(phi)*cos(psi);
             -sin(theta),          sin(phi)*cos(theta),                            cos(phi)*cos(theta) ];
    pos_dot = R_b2e * vel_b;
    
    tt = tan(theta); ct = cos(theta); 
    if ct >= 0, ct = max(ct, 0.001); else, ct = min(ct, -0.001); end
    
    euler_dot = [ rates(1) + (rates(2)*sin(phi) + rates(3)*cos(phi)) * tt;
                  rates(2)*cos(phi) - rates(3)*sin(phi);
                 (rates(2)*sin(phi) + rates(3)*cos(phi)) / ct ];
                 
    % 6. ĐÓNG GÓI AN TOÀN
    % Nếu có vector nào bị phình lên 4x1 do cắm sai dây, Coder sẽ ném lỗi ngay tại 4 dòng này.
    dx(1:3)   = pos_dot;
    dx(4:6)   = acc_b;
    dx(7:9)   = euler_dot;
    dx(10:12) = rate_dot;
end
